simulink model "srikri_dab_try"  (R2022b)
settings: Solver=VariableStepAuto  StartTime=0.0  StopTime=2e-2  RelTol=1e-3
libraries: spsDiodeLib x8, spsIGBTLib x8, spsCurrentMeasurementLib x3, spsStairGeneratorLib x3, spsControlledVoltageSourceLib x2, spsMultimeterLib x2, ee_lib x1, spsLinearTransformerLib x1, slpidlib x1, spsSaturableTransformerLib x1, spsSeriesRLCBranchLib x1, spsVoltageMeasurementLib x1
settings Model: Creator=srikr  LastModifiedBy=srikri

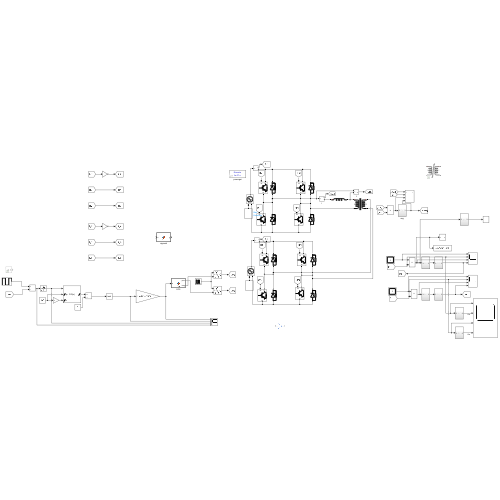
[thumbnail: Simulink's stored preview of the top-level diagram]
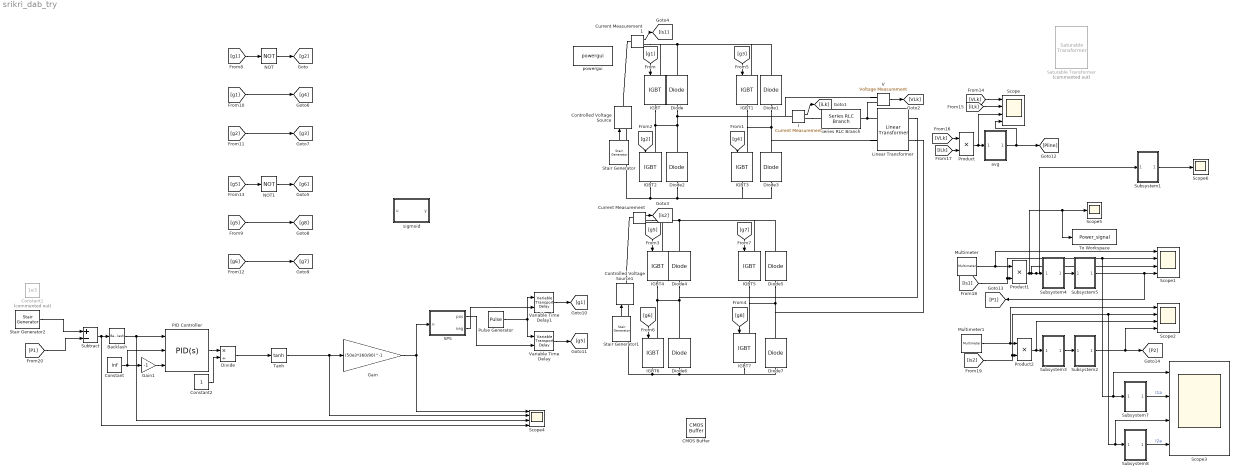
== system srikri_dab_try ==
  Backlash : Backlash  BacklashWidth=0
  CMOS Buffer : ee_lib/Integrated Circuits/Logic/CMOS Buffer  V_IL=2 V  V_IH=3 V  C_IN=5 pF  output_type=ee.enum.ic.outputType.linear  V_OL=0 V  V_OH=5 V  V_CC=5 V  V_meas=5 V  R_OUT=25 Ohm  R_OH=[25, 250] Ohm  I_OH=63 mA  R_OL=[30, 800] Ohm  I_OL=-45 mA  Delay=25 ns  Ron=5 Ohm  Vf=0.6 V  output_state=ee.enum.ic.initialState.low
      settings: InternalSimscapePortConfiguration="{\"Bottom\":[],\"Left\":[{\"id\":\"A\",\"label\":\"\",\"type\":\"foundation.electrical.electrical\"}],\"Right\":[{\"id\":\"J\",\"label\":\"\",\"type\":\"foundation.electrical.electrical\"}],\"Top\":[]}"
  Constant : Constant  Value=inf
  Constant1 : Constant  Commented=on  Value=1e3
  Constant2 : Constant
  Controlled Voltage Source : spsControlledVoltageSourceLib/Controlled Voltage Source  Initialize=on  Source_Type=AC  Amplitude=0  Phase=0  Frequency=0  Measurements=Voltage
  Controlled Voltage Source1 : spsControlledVoltageSourceLib/Controlled Voltage Source  Initialize=on  Source_Type=AC  Amplitude=0  Phase=0  Frequency=0  Measurements=Voltage
  Current Measurement : spsCurrentMeasurementLib/Current Measurement  PhasorSimulation=off  OutputType=Complex  PSBequivalent=0
  Current Measurement1 : spsCurrentMeasurementLib/Current Measurement  PhasorSimulation=off  OutputType=Complex  PSBequivalent=0
  Diode{,1..7} (8 alike) : spsDiodeLib/Diode  Ron=0.001  Lon=0  Vf=0.8  IC=0  UseSnubber=0  Rs=500  Cs=250e-9  Measurements=off
  Divide : Product  Inputs=*/
  Gain : Gain  Gain=(50e3*360/90)^-1
  Gain1 : Gain  Gain=-1
  I : spsCurrentMeasurementLib/Current Measurement  PhasorSimulation=off  OutputType=Complex  PSBequivalent=0
  IGBT{,1..7} (8 alike) : spsIGBTLib/IGBT  Ron=0.001  Lon=0  Vf=1  Tf=1e-6  Tt=2e-6  IC=0  Rs=1e5  Cs=inf  Measurements=off
  Linear Transformer : spsLinearTransformerLib/Linear Transformer  UNITS=SI  NominalPower=[ 250e6 30e3 ]  winding1=[200 0 0]  winding2=[100 0 0]  ThreeWindings=off  winding3=[3.15e+05 0.7938 0.084225]  RmLm=[30e3 1e-3]  Measurements=All voltages and currents  DataType=on
  Multimeter : spsMultimeterLib/Multimeter  L=11  sel=4  yselected={}  Gain=1  OutputType=Complex  PlotAtSimulationStop=off  PhasorSimulation=off
  Multimeter1 : spsMultimeterLib/Multimeter  L=11  sel=4  yselected={}  Gain=1  OutputType=Complex  PlotAtSimulationStop=off  PhasorSimulation=off
  NOT : Logic  Operator=NOT  IconShape=distinctive  AllPortsSameDT=off  OutDataTypeStr=boolean
  NOT1 : Logic  Operator=NOT  IconShape=distinctive  AllPortsSameDT=off  OutDataTypeStr=boolean
  PID Controller : slpidlib/PID Controller  Controller=PID  Form=Parallel  TimeDomain=Continuous-time  UseExternalTs=off  SampleTime=-1  IntegratorMethod=Forward Euler  FilterMethod=Forward Euler  ControllerParametersSource=internal  P=1e-1  I=0  UseKiTs=off  D=0  N=100  UseFilter=on  TunerSelectOption=Frequency Response Based  InitialConditionSource=internal  InitialConditionForIntegrator=0  InitialConditionForFilter=0  DifferentiatorICPrevScaledInput=0  ExternalReset=none  TrackingMode=off  Kt=1  LimitOutput=on  SatLimitsSource=external  UpperSaturationLimit=1e3  LowerSaturationLimit=-1e3  LinearizeAsGain=on  AntiWindupMode=none  Kb=1  LimitIntegrator=off  UpperIntegratorSaturationLimit=inf  LowerIntegratorSaturationLimit=-inf  POutMin=[]  POutMax=[]  IOutMin=[]  IOutMax=[]  DOutMin=[]  DOutMax=[]  NOutMin=[]  NOutMax=[]  SumOutMin=[]  SumOutMax=[]  SaturationOutMin=[]  SaturationOutMax=[]  PParamMin=[]  PParamMax=[]  IParamMin=[]  IParamMax=[]  DParamMin=[]  DParamMax=[]  NParamMin=[]  NParamMax=[]  KbParamMin=[]  KbParamMax=[]  KtParamMin=[]  KtParamMax=[]  KbOutMin=[]  KbOutMax=[]  KtOutMin=[]  KtOutMax=[]  IntegratorOutMin=[]  IntegratorOutMax=[]  FilterOutMin=[]  FilterOutMax=[]  SumI1OutMin=[]  SumI1OutMax=[]  SumI2OutMin=[]  SumI2OutMax=[]  SumI3OutMin=[]  SumI3OutMax=[]  SumI4OutMin=[]  SumI4OutMax=[]  SumDOutMin=[]  SumDOutMax=[]  DifferentiatorOutMin=[]  DifferentiatorOutMax=[]  FilterDiffOutCoefMin=[]  FilterDiffOutCoefMax=[]  ReciprocalOutMin=[]  ReciprocalOutMax=[]  SumDenOutMin=[]  SumDenOutMax=[]  SumNumOutMin=[]  SumNumOutMax=[]  DivideOutMin=[]  DivideOutMax=[]  UdiffTsProdOutMin=[]  UdiffTsProdOutMax=[]  NTsProdOutMin=[]  NTsProdOutMax=[]  UintegralTsProdOutMin=[]  UintegralTsProdOutMax=[]  UngainTsProdOutMin=[]  UngainTsProdOutMax=[]  ClampingZeroOutDataTypeStr=Inherit: Inherit via back propagation  ClampingZeroOutMin=[]  ClampingZeroOutMax=[]  FilterDenConstantOutDataTypeStr=Inherit: Inherit via back propagation  FilterDenConstantOutMin=[]  FilterDenConstantOutMax=[]  PCopyOutDataTypeStr=Inherit: Inherit via back propagation  PCopyOutMin=[]  PCopyOutMax=[]  NCopyOutDataTypeStr=Inherit: Inherit via back propagation  NCopyOutMin=[]  NCopyOutMax=[]  IntegratorContinuousStateAttributes=''  IntegratorStateMustResolveToSignalObject=off  IntegratorRTWStateStorageClass=Auto  FilterContinuousStateAttributes=''  FilterStateMustResolveToSignalObject=off  FilterRTWStateStorageClass=Auto  ParallelPVariant=InternalParameters  IdealPVariant=Disabled  IVariant=InternalParameters  DVariant=InternalParameters  IntegratorVariant=Continuous  SatVariant=External  AWVariant=Passthrough  PCopyVariant=Disabled  TRVariant=Disabled  FdbkBlocksVariant=Forward  IdealPFdbkVariant=Disabled  SatFdbkVariant=Disabled  DerivativeFilterVariant=ContFilter  NVariant=InternalParameters  NCopyVariant=Disabled  FilterICVariant=InternalICsFilter  IntegratorICVariant=InternalICs  ExternalResetVariant=Disabled  TRSumVariant=Passthrough  SumFdbkVariant=Disabled  SumVariant=Sum_PID  TsampFilterVariant=InternalTs  TsampNgainVariant=Passthrough  TsampIntegralVariant=Passthrough  ExternalSaturationOutDataTypeStr=Inherit: Same as second input
  Product : Product
  Product1 : Product
  Product2 : Product
  Pulse Generator : DiscretePulseGenerator  PulseType=Time based  Period=1/50e3  PulseWidth=50
  SPS : MATLAB Function  TreatAsAtomicUnit=on
  Saturable Transformer : spsSaturableTransformerLib/Saturable Transformer  Commented=on  ThreeWindings=off  Hysteresis=off  DataFile='hysteresis.mat'  Measurements=All measurements (V I Flux)  UNITS=SI  NominalPower=[250e6 60]  Winding1=[200 0 0]  Winding2=[100 0 0]  Winding3=[3.15e+05 0.7938 0.084225]  Saturation=[0 0;1 100;]  CoreLoss=25e3  BreakLoop=off  DiscreteSolver=Trapezoidal iterative  DataType=on  InitialFlux=0  TransfoNumber=1
      settings: LibrarySourceBlock=sps_lib/Power Grid Elements/Saturable Transformer
  Scope{,1..4} (5 alike) : Scope  NumInputPorts=4
  Scope5 : Scope
  Scope6 : Scope
  Series RLC Branch : spsSeriesRLCBranchLib/Series RLC Branch  LConnTagsString=__new0  RConnTagsString=__new0  BranchType=L  Resistance=1  Inductance=50e-6  SetiL0=off  InitialCurrent=0  Capacitance=1e-6  Setx0=off  InitialVoltage=0  Measurements=Branch voltage and current
  Stair Generator : spsStairGeneratorLib/Stair Generator  t=[0,0.5]*2e-2  e=[100, 100]  Ts=0
  Stair Generator1 : spsStairGeneratorLib/Stair Generator  t=[0,0.25]*2e-2  e=[100, 100]  Ts=0
  Stair Generator2 : spsStairGeneratorLib/Stair Generator  t=[0:.25:1]*2e-2  e=[0,1e3,0,1e3,0.5e3]  Ts=0
  Subsystem1 : Subsystem
  Subsystem2 : Subsystem
  Subsystem3 : Subsystem
  Subsystem4 : Subsystem
  Subsystem5 : Subsystem
  Subsystem7 : Subsystem
  Subsystem8 : Subsystem
  Subtract : Sum  Inputs=+-
  Tanh : Trigonometry  Operator=tanh
  To Workspace : ToWorkspace  VariableName=Power_signal  SaveFormat=Timeseries  SampleTime=-1
  V : spsVoltageMeasurementLib/Voltage Measurement  PhasorSimulation=off  OutputType=Complex  PSBequivalent=0
  Variable Time Delay : VariableTransportDelay  MaximumDelay=10
  Variable Time Delay1 : VariableTransportDelay  MaximumDelay=10
  avg : Subsystem
  powergui : sps_lib/powergui  Priority=1  SimulationMode=Discrete  SampleTime=1e-7  frequency=60  Iterations=50  frequencyindice=0  Pbase=100e6  ErrMax=1e-4  UnitsV=kV  UnitsW=MW  buscounter=0  FunctionMessages=off  echomessages=off  EnableUseOfTLC=off  CurrentSourceSwitches=off  DisableSnubberDevices=off  DisableRonSwitches=off  DisableVfSwitches=off  DisplayEquations=off  AutomaticDiscreteSolvers=off  SolverType=Tustin/Backward Euler (TBE)  Interpol=off  ExternalGateDelay=off  methode=off  Ts=100  x0status=blocks  SPID=on  SwTol=0  HookPort=off  NonlinearTolerance=1e-4  nMaxIteration=100  ContinueOnMaxIteration=off  RestoreLinks=warning  ResistiveCurrentMeasurement=off  Frange=[0:2:500]  Ylog=off  Xlog=on  ShowGrid=off  save=off  variable=ZData  structure=0  ZoomFFT=off  StartTime=0.0  cycles=1  DisplayStyle=1  fundamental=60  FreqAxis=off  MaxFrequency=1000  frequencyindicesteady=1  RmsSteady=1  display=off
  sigmoid : MATLAB Function  TreatAsAtomicUnit=on
  wires:
  [g3] -> IGBT1/1
  [g1] -> IGBT/1
  [g2] -> IGBT2/1
  [g4] -> IGBT3/1
  [g8] -> IGBT7/1
  [g6] -> IGBT6/1
  [g7] -> IGBT5/1
  [g5] -> IGBT4/1
  [g1] -> NOT/1
  NOT/1 -> [g2]
  [g1] -> [g4]
  [g2] -> [g3]
  [g5] -> NOT1/1
  [g5] -> [g8]
  [g6] -> [g7]
  NOT1/1 -> [g6]
  Pulse Generator/1 -> Variable Time Delay1/1, Variable Time Delay/1
  Variable Time Delay/1 -> [g5]
  Gain/1 -> SPS/1(u), Scope4/1
  I/1 -> [iLk]
  V/1 -> [VLk]
  [VLk] -> Scope/1
  [iLk] -> Scope/2
  Product/1 -> Scope/3, avg/1(In1)
  [VLk] -> Product/1
  [iLk] -> Product/2
  avg/1(Out1) -> [Pline], Scope/4
  Current Measurement/1 -> [is2]
  Multimeter/1 -> Product1/1, Scope1/1
  [is1] -> Scope3/1, Subsystem7/1(In1), Scope1/2, Product1/2
  Current Measurement1/1 -> [is1]
  [is2] -> Scope3/3, Subsystem8/1(In1), Scope2/2, Product2/2
  Product2/1 -> Subsystem3/1(In1), Scope2/3
  Multimeter1/1 -> Scope2/1, Product2/1
  Subsystem3/1(Out1) -> Subsystem2/1(In1)
  Stair Generator/1 -> Controlled Voltage Source/1
  Subsystem7/1(Out1) -> Scope3/2  "I1a"
  Subsystem8/1(Out1) -> Scope3/4  "I2a"
  Stair Generator1/1 -> Controlled Voltage Source1/1
  Subtract/1 -> Scope4/4, Backlash/1
  Stair Generator2/1 -> Subtract/1
  [P1] -> Subtract/2
  Subsystem2/1(Out1) -> [P2], Scope2/4
  Subsystem1/1(Out1) -> Scope6/1
  Product1/1 -> To Workspace/1, Scope5/1, Subsystem1/1(In1), Subsystem4/1(In1), Scope1/3
  Variable Time Delay1/1 -> [g1]
  SPS/1(pos) -> Variable Time Delay/2
  SPS/2(neg) -> Variable Time Delay1/2
  Backlash/1 -> Scope4/3, PID Controller/1
  Constant/1 -> PID Controller/2, Gain1/1
  Gain1/1 -> PID Controller/3
  PID Controller/1 -> Divide/1
  Divide/1 -> Tanh/1
  Subsystem4/1(Out1) -> Subsystem5/1(In1)
  Constant2/1 -> Divide/2
  Tanh/1 -> Gain/1, Scope4/2
  Subsystem5/1(Out1) -> Scope1/4, [P1]
  connections:
  Diode1/LConn1 -- Linear Transformer/LConn2 -- Diode3/RConn1 -- IGBT1/RConn1 -- IGBT3/LConn1
  Diode/RConn1 -- Current Measurement1/RConn1 -- IGBT/LConn1 -- IGBT1/LConn1 -- Diode1/RConn1
  IGBT2/RConn1 -- Controlled Voltage Source/LConn1 -- Diode3/LConn1 -- IGBT3/RConn1 -- Diode2/LConn1
  IGBT2/LConn1 -- IGBT/RConn1 -- I/LConn1 -- V/LConn1 -- Diode/LConn1 -- Diode2/RConn1
  IGBT6/RConn1 -- Controlled Voltage Source1/LConn1 -- Diode7/LConn1 -- IGBT7/RConn1 -- Diode6/LConn1
  Diode5/LConn1 -- Linear Transformer/RConn2 -- Diode7/RConn1 -- IGBT5/RConn1 -- IGBT7/LConn1
  Diode4/RConn1 -- Current Measurement/RConn1 -- IGBT4/LConn1 -- Diode5/RConn1 -- IGBT5/LConn1
  IGBT6/LConn1 -- Diode6/RConn1 -- Linear Transformer/RConn1 -- Diode4/LConn1 -- IGBT4/RConn1
  Series RLC Branch/RConn1 -- V/LConn2 -- Linear Transformer/LConn1
  I/RConn1 -- Series RLC Branch/LConn1
  Controlled Voltage Source1/RConn1 -- Current Measurement/LConn1
  Controlled Voltage Source/RConn1 -- Current Measurement1/LConn1

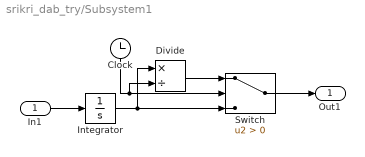
== system srikri_dab_try/Subsystem1 ==
  In1 : Inport
  Clock : Clock
  Divide : Product  Inputs=*/
  Integrator : Integrator
  Switch : Switch  Criteria=u2 > Threshold  SaturateOnIntegerOverflow=off  InputSameDT=off
  Out1 : Outport
  wires:
  Divide/1 -> Switch/1
  Integrator/1 -> Switch/3, Divide/1
  Clock/1 -> Switch/2, Divide/2
  In1/1 -> Integrator/1
  Switch/1 -> Out1/1

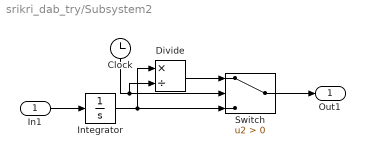
== system srikri_dab_try/Subsystem2 ==
  In1 : Inport
  Clock : Clock
  Divide : Product  Inputs=*/
  Integrator : Integrator
  Switch : Switch  Criteria=u2 > Threshold  SaturateOnIntegerOverflow=off  InputSameDT=off
  Out1 : Outport
  wires:
  Divide/1 -> Switch/1
  Integrator/1 -> Switch/3, Divide/1
  Clock/1 -> Switch/2, Divide/2
  In1/1 -> Integrator/1
  Switch/1 -> Out1/1

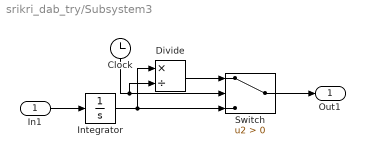
== system srikri_dab_try/Subsystem3 ==
  In1 : Inport
  Clock : Clock
  Divide : Product  Inputs=*/
  Integrator : Integrator
  Switch : Switch  Criteria=u2 > Threshold  SaturateOnIntegerOverflow=off  InputSameDT=off
  Out1 : Outport
  wires:
  Divide/1 -> Switch/1
  Integrator/1 -> Switch/3, Divide/1
  Clock/1 -> Switch/2, Divide/2
  In1/1 -> Integrator/1
  Switch/1 -> Out1/1

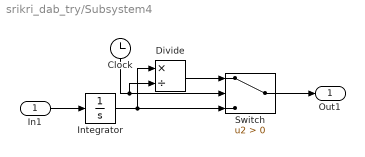
== system srikri_dab_try/Subsystem4 ==
  In1 : Inport
  Clock : Clock
  Divide : Product  Inputs=*/
  Integrator : Integrator
  Switch : Switch  Criteria=u2 > Threshold  SaturateOnIntegerOverflow=off  InputSameDT=off
  Out1 : Outport
  wires:
  Divide/1 -> Switch/1
  Integrator/1 -> Switch/3, Divide/1
  Clock/1 -> Switch/2, Divide/2
  In1/1 -> Integrator/1
  Switch/1 -> Out1/1

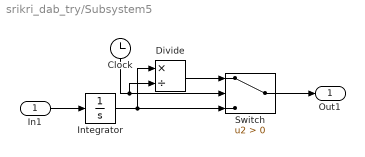
== system srikri_dab_try/Subsystem5 ==
  In1 : Inport
  Clock : Clock
  Divide : Product  Inputs=*/
  Integrator : Integrator
  Switch : Switch  Criteria=u2 > Threshold  SaturateOnIntegerOverflow=off  InputSameDT=off
  Out1 : Outport
  wires:
  Divide/1 -> Switch/1
  Integrator/1 -> Switch/3, Divide/1
  Clock/1 -> Switch/2, Divide/2
  In1/1 -> Integrator/1
  Switch/1 -> Out1/1

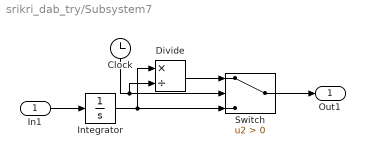
== system srikri_dab_try/Subsystem7 ==
  In1 : Inport
  Clock : Clock
  Divide : Product  Inputs=*/
  Integrator : Integrator
  Switch : Switch  Criteria=u2 > Threshold  SaturateOnIntegerOverflow=off  InputSameDT=off
  Out1 : Outport
  wires:
  Divide/1 -> Switch/1
  Integrator/1 -> Switch/3, Divide/1
  Clock/1 -> Switch/2, Divide/2
  In1/1 -> Integrator/1
  Switch/1 -> Out1/1

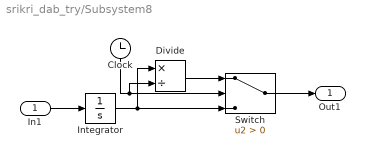
== system srikri_dab_try/Subsystem8 ==
  In1 : Inport
  Clock : Clock
  Divide : Product  Inputs=*/
  Integrator : Integrator
  Switch : Switch  Criteria=u2 > Threshold  SaturateOnIntegerOverflow=off  InputSameDT=off
  Out1 : Outport
  wires:
  Divide/1 -> Switch/1
  Integrator/1 -> Switch/3, Divide/1
  Clock/1 -> Switch/2, Divide/2
  In1/1 -> Integrator/1
  Switch/1 -> Out1/1

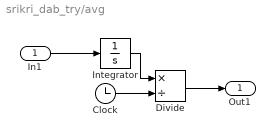
== system srikri_dab_try/avg ==
  In1 : Inport
  Clock : Clock
  Divide : Product  Inputs=*/
  Integrator : Integrator
  Out1 : Outport
  wires:
  Divide/1 -> Out1/1
  Clock/1 -> Divide/2
  Integrator/1 -> Divide/1
  In1/1 -> Integrator/1

== matlab function srikri_dab_try/sigmoid ==
  data: u input; y output
function y = fcn(u)

y = 1/(1 + exp(-u));

== matlab function srikri_dab_try/SPS ==
  data: u input; pos output; neg output
function [pos,neg] = fcn(u)

if u>=0
    pos = u;
    neg = 0;
else
    neg = u;
    pos = 0;
end
